simulink model "Berechnung_Generatormoment"  (R2022b)
settings: Solver=VariableStepAuto  StartTime=0.0  StopTime=10.0  RelTol=1e-3
undefined symbols (not defined in the file): beta_array, CQ_entries, lambda_array, param_const
settings Model: Creator=Sebastian  LastModifiedBy=Sebastian

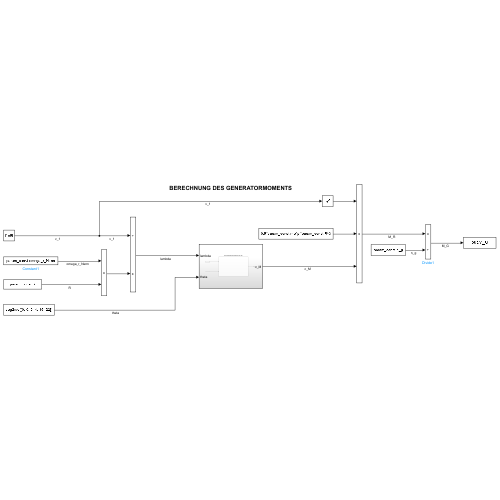
[thumbnail: Simulink's stored preview of the top-level diagram]
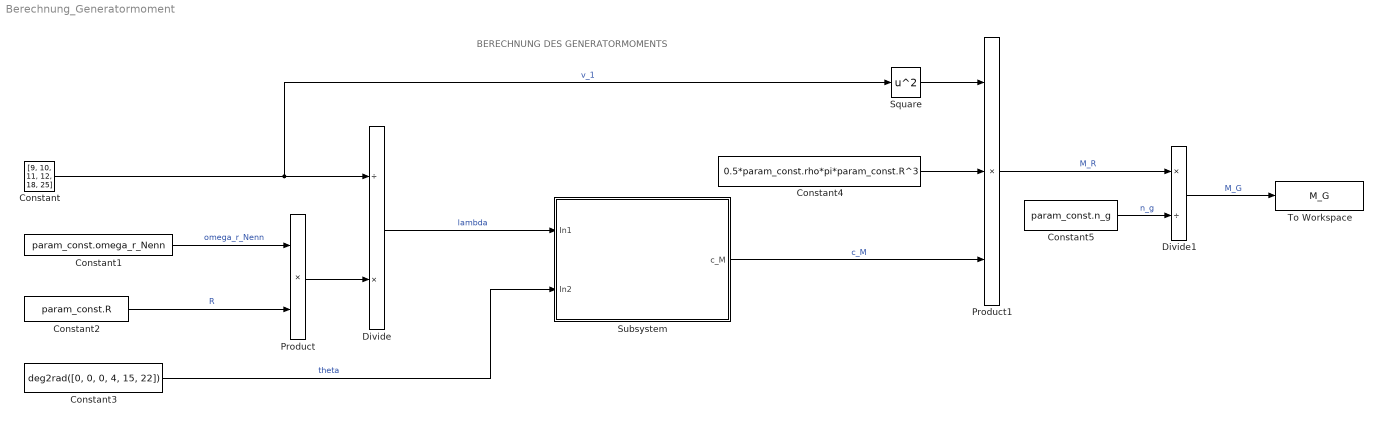
== system Berechnung_Generatormoment ==
  note: BERECHNUNG DES GENERATORMOMENTS
  Constant : Constant  Value=[9, 10, 11, 12, 18, 25]
  Constant1 : Constant  Value=param_const.omega_r_Nenn
  Constant2 : Constant  Value=param_const.R
  Constant3 : Constant  Value=deg2rad([0, 0, 0, 4, 15, 22])
  Constant4 : Constant  Value=0.5*param_const.rho*pi*param_const.R^3
  Constant5 : Constant  Value=param_const.n_g
  Divide : Product  Inputs=/*
  Divide1 : Product  Inputs=*/
  Product : Product
  Product1 : Product  Inputs=3
  Square : Math  Operator=square
  Subsystem : Subsystem
  To Workspace : ToWorkspace  VariableName=M_G  SaveFormat=Timeseries  SampleTime=-1
  wires:
  Constant1/1 -> Product/1  "omega_r_Nenn"
  Constant2/1 -> Product/2  "R"
  Product/1 -> Divide/2
  Constant/1 -> Square/1, Divide/1  "v_1"
  Divide/1 -> Subsystem/1(In1)  "lambda"
  Constant3/1 -> Subsystem/2(In2)  "theta"
  Subsystem/1(c_M) -> Product1/3  "c_M"
  Constant4/1 -> Product1/2
  Product1/1 -> Divide1/1  "M_R"
  Constant5/1 -> Divide1/2  "n_g"
  Divide1/1 -> To Workspace/1  "M_G"
  Square/1 -> Product1/1

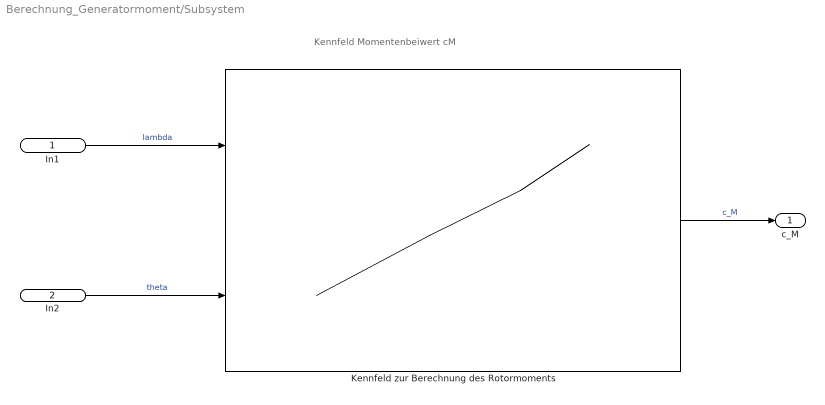
== system Berechnung_Generatormoment/Subsystem ==
  note: Kennfeld Momentenbeiwert cM
  In1 : Inport
  In2 : Inport  Port=2
  Kennfeld zur Berechnung des Rotormoments : Lookup_n-D  BreakpointsForDimension1=lambda_array  BreakpointsForDimension2=beta_array  Table=CQ_entries  InternalRulePriority=Speed  RndMeth=Simplest
      settings: InputPortMap=u0,u1
  c_M : Outport
  wires:
  Kennfeld zur Berechnung des Rotormoments/1 -> c_M/1  "c_M"
  In1/1 -> Kennfeld zur Berechnung des Rotormoments/1  "lambda"
  In2/1 -> Kennfeld zur Berechnung des Rotormoments/2  "theta"
